simulink model "OUmControladorDiscreto"  (R2018a)
settings: Solver=VariableStepAuto  StartTime=0.0  StopTime=10.0  RelTol=1e-3
values from neighbouring files (symbols this model uses):
  Td = 1    [pid_iterativo.m]
  Ti = 42    [pid_iterativo.m]
undefined symbols (not defined in the file or in its folder): Kc
settings Model: Creator=vittorfp  LastModifiedBy=vittorfp

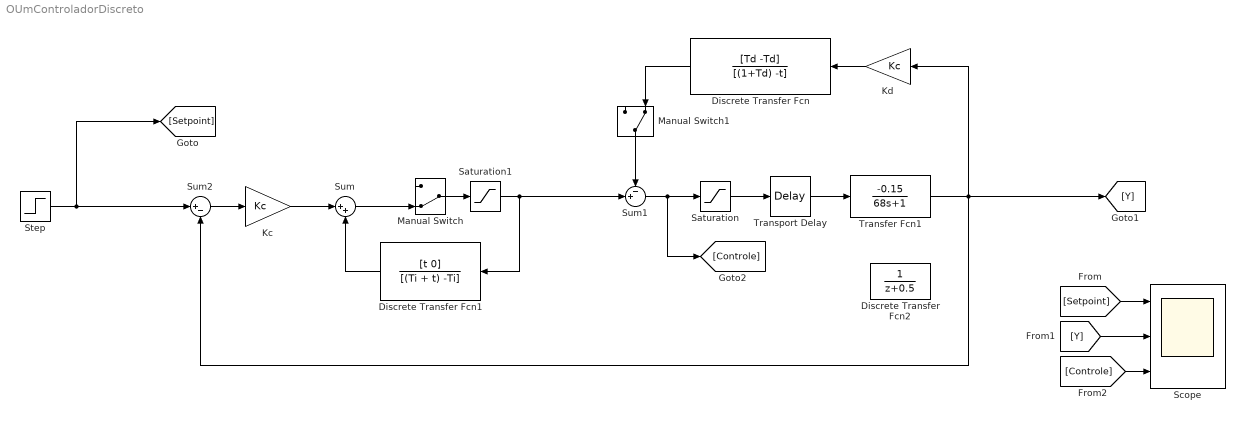
== system OUmControladorDiscreto ==
  Discrete Transfer Fcn : DiscreteTransferFcn  Numerator=[Td -Td]  Denominator=[(1+Td) -t]
  Discrete Transfer Fcn1 : DiscreteTransferFcn  Numerator=[t 0]  Denominator=[(Ti + t) -Ti]
  Discrete Transfer Fcn2 : DiscreteTransferFcn
  Kc : Gain  Gain=Kc
  Kd : Gain  Gain=Kc
  Manual Switch : ManualSwitch  CurrentSetting=0
  Manual Switch1 : ManualSwitch  CurrentSetting=0
  Saturation : Saturate  UpperLimit=10225  LowerLimit=-23200
  Saturation1 : Saturate  UpperLimit=10225  LowerLimit=-23200
  Scope : Scope  NumInputPorts=3
  Step : Step  After=2000  SampleTime=0
  Sum : Sum  Inputs=|++
  Sum1 : Sum  Inputs=-+|
  Sum2 : Sum  Inputs=|+-
  Transfer Fcn1 : TransferFcn  Numerator=[-0.15]  Denominator=[68 1]
  Transport Delay : TransportDelay  DelayTime=19
  wires:
  Manual Switch1/1 -> Sum1/1
  [Y] -> Scope/2
  Sum2/1 -> Kc/1
  Sum/1 -> Manual Switch/2
  Discrete Transfer Fcn1/1 -> Sum/2
  Manual Switch/1 -> Saturation1/1
  Kd/1 -> Discrete Transfer Fcn/1
  Transfer Fcn1/1 -> [Y], Kd/1, Sum2/2
  Kc/1 -> Sum/1
  [Setpoint] -> Scope/1
  [Controle] -> Scope/3
  Transport Delay/1 -> Transfer Fcn1/1
  Saturation/1 -> Transport Delay/1
  Step/1 -> Sum2/1, [Setpoint]
  Sum1/1 -> [Controle], Saturation/1
  Discrete Transfer Fcn/1 -> Manual Switch1/2
  Saturation1/1 -> Discrete Transfer Fcn1/1, Sum1/2
